simulink model "Vision_Algorithm"  (R2018a)
settings: Solver=FixedStepAuto  StartTime=0.0  StopTime=inf  RelTol=1e-3  EnableMultiTasking=on
libraries: simulink x1
settings Model: SimulationMode=external  Creator=cdsouza  LastModifiedBy=scastro
settings SolverCC: PositivePriorityOrder=on
settings OptimizationCC: EnhancedBackFolding=on  PassReuseOutputArgsAs=Individual arguments  MaxStackSize=64  OptimizeBlockOrder=speed  DifferentSizesBufferReuse=on  OptimizationCustomize=off
settings DebuggingCC: ParameterTunabilityLossMsg=error
settings HardwareCC: ProdBitPerPointer=32  ProdBitPerSizeT=32  ProdBitPerPtrDiffT=32  ProdLargestAtomicInteger=Long  ProdLargestAtomicFloat=Double  ProdWordSize=32  ProdHWDeviceType=ARM Compatible->ARM Cortex
settings SFSimCC: MATLABDynamicMemAlloc=off
settings RTWCC: SystemTargetFile=ert.tlc  HardwareBoard=Raspberry Pi  TLCOptions="-aInlineSetEventsForThisBaseRateFcn=TLC_FALSE -aSuppressMultiTaskScheduler=TLC_FALSE  -aRateBasedStepFcn=0"  TemplateMakefile=ert_default_tmf  GenerateReport=on  Toolchain=GNU GCC Raspberry Pi  BuildConfiguration=Faster Runs  IncludeHyperlinkInReport=on  LaunchReport=on  GenerateTraceInfo=on  GenerateTraceReport=on  GenerateTraceReportSl=on  GenerateTraceReportSf=on  GenerateTraceReportEml=on
settings CodeAppCC: ForceParamTrailComments=on  IgnoreCustomStorageClasses=off  OperatorAnnotations=on  SimulinkDataObjDesc=on  SFDataObjDesc=on  InsertBlockDesc=on
settings ERTTargetCC: SupportVariableSizeSignals=on

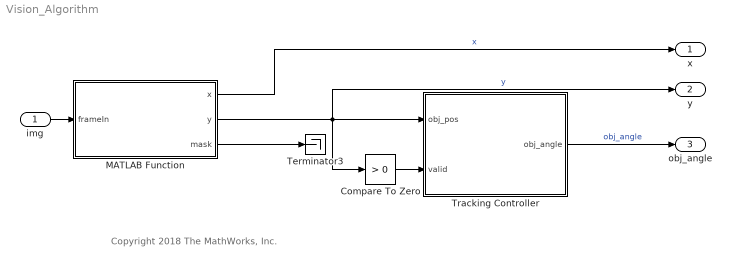
== system Vision_Algorithm ==
  note: Copyright 2018 The MathWorks, Inc.
  img : Inport  OutDataTypeStr=uint8  PortDimensions=[320 240 3]  SampleTime=[0.050000000000000003,0]
  Compare To Zero : simulink/Logic and Bit Operations/Compare To Zero  relop=>  OutDataTypeStr=boolean  ZeroCross=off
  MATLAB Function : MATLAB Function  TreatAsAtomicUnit=on
  Terminator3 : Terminator
  Tracking Controller : Stateflow chart  TreatAsAtomicUnit=on
  x : Outport  OutDataTypeStr=double  PortDimensions=1  SampleTime=[0.050000000000000003,0]
  y : Outport  Port=2  OutDataTypeStr=double  PortDimensions=1  SampleTime=[0.050000000000000003,0]
  obj_angle : Outport  Port=3  OutDataTypeStr=double  PortDimensions=1  SampleTime=[0.050000000000000003,0]
  wires:
  MATLAB Function/3(mask) -> Terminator3/1
  MATLAB Function/1(x) -> x/1  "x"
  MATLAB Function/2(y) -> Tracking Controller/1(obj_pos), Compare To Zero/1, y/1  "y"
  Compare To Zero/1 -> Tracking Controller/2(valid)
  img/1 -> MATLAB Function/1(frameIn)
  Tracking Controller/1(obj_angle) -> obj_angle/1  "obj_angle"

== stateflow chart Vision_Algorithm/Tracking Controller ==
  settings: sampleTime=1/15
  state dir = setDir(position) [function]
    (default) -> (junction 70)
    (junction 70) -> (junction 74) [order 1] : [position > 160]
    (junction 70) -> (junction 76) [order 2] : {dir = -1;}
    (junction 74) -> (junction 78) : {dir = 1;}
    (junction 78) -> (junction 76)
    (junction 76) -> (junction 86)
  state Tracking
    entry, during:
    obj_angle = objAngle(obj_pos);
    direction = setDir(obj_pos);
  state Waiting
    entry:
    i = 0;
    during:
    i = i + 1;
  state Seeking
    Seeking -> (junction 33) [order 1]
    (junction 33) -> (junction 40) [order 2]
    (junction 33) -> (junction 37) [order 1] : [direction==1]
    (junction 37) -> (junction 43) [order 2] : {direction=-1;}
    (junction 40) -> (junction 47) [order 2] : {direction=1;}
    (junction 37) -> (junction 43) [order 1] : [obj_angle < MAX_ANGLE]
        | {obj_angle = obj_angle + 10;}
    (junction 40) -> (junction 47) [order 1] : [obj_angle>-MAX_ANGLE]
        | {obj_angle = obj_angle - 10;}
    (junction 47) -> (junction 61)
    (junction 43) -> (junction 61)
  (default) -> Tracking
  Tracking -> Waiting : [~valid]
  Waiting -> Tracking [order 2] : [valid]
  Waiting -> Seeking [order 1] : [i>10]
  Seeking -> Tracking [order 1] : [valid]
  data: position function_input double; dir function_output double; pos function_input double; a function_output double; obj_pos input double; MAX_ANGLE local double =90; valid input; i local double; obj_angle output double; direction local double
  function a = objAngle(pos):
    | function a = objAngle(pos)
    | 
    | % a = atand((pos-200)/5000);
    | deadZone = 0.2;
    | 
    | a =(pos - 160)/160;
    | 
    | if abs(a)<(deadZone/2)
    |    a=0;
    | end
    | 
    | 
    | end

== matlab function Vision_Algorithm/MATLAB Function ==
  data: x output; frameIn input uint8 size=[320 240 3]; y output; mask output size=[320 240]
function [x,y,mask] = detectROI(frameIn)
%#Codegen 

% This funtcion thresholds the image based on threshold values submitted by
% the user

%% Setup the detector and initialize variables
persistent detector 
if isempty(detector)
    detector = vision.BlobAnalysis('BoundingBoxOutputPort',false,...
        'AreaOutputPort',false,'MinimumBlobArea',300, ...
        'MajorAxisLengthOutputPort',true,'MaximumCount', 10);
end
x = 0;
y = 0;
threshold = [107.00 225.00; 85.000 120.000; 82.000 121.000];

%% Threshold the image
frameIn = rgb2ycbcr(frameIn);
mask = (frameIn (:,:,1) >= threshold(1,1))& (frameIn (:,:,1) <= threshold(1,2))&...
    (frameIn (:,:,2) >= threshold(2,1))& (frameIn (:,:,2) <= threshold(2,2))&...
    (frameIn (:,:,3) >= threshold(3,1))& (frameIn (:,:,3) <= threshold(3,2));

[centroid,majorAxis] = detector(mask);


if ~isempty(majorAxis)
% Identify Largest Blob
    [~,mIdx] = max(majorAxis);
    C = centroid(mIdx,:);
    x = double(C(1));
    y = double(C(2));

end 

end
